simulink model "ModelMCC"  (R2018a)
settings: Solver=VariableStepAuto  StartTime=0.0  StopTime=10  RelTol=1e-3
undefined symbols (not defined in the file): A, f, J, K, L, N, R
libraries: simulink x1, powerlib x1
settings Model: Creator=Utilisateur  LastModifiedBy=Utilisateur

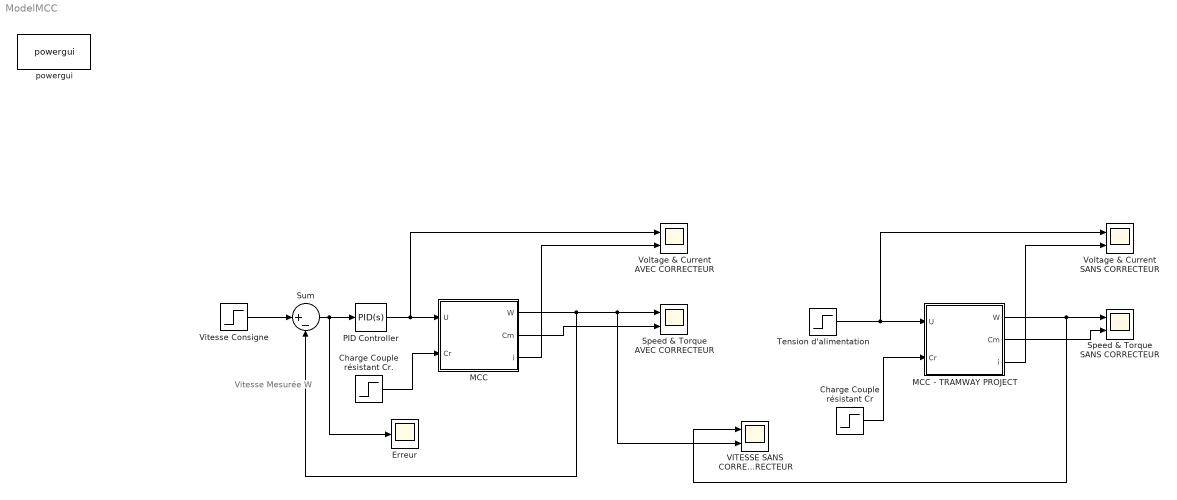
== system ModelMCC ==
  note: Vitesse Mesurée
      | W
  Charge Couple résistant Cr : Step  Time=5  After=30  SampleTime=0
  Charge Couple résistant Cr. : Step  Time=5  After=30  SampleTime=0
  Erreur : Scope
  MCC : Subsystem
  MCC - TRAMWAY PROJECT : Subsystem
  PID Controller : simulink/Continuous/PID Controller  Controller=PID  TimeDomain=Continuous-time  SampleTime=-1  IntegratorMethod=Forward Euler  FilterMethod=Forward Euler  Form=Parallel  UseFilter=on  ControllerParametersSource=internal  P=23.9565323270696  I=104.937795909472  D=-0.463662749906511  N=7.82954211558253  InitialConditionSource=internal  InitialConditionForIntegrator=0  InitialConditionForFilter=0  ExternalReset=none  LimitOutput=off  UpperSaturationLimit=inf  LowerSaturationLimit=-inf  LinearizeAsGain=on  AntiWindupMode=none  Kb=1  TrackingMode=off  Kt=1  PParamMin=[]  PParamMax=[]  IParamMin=[]  IParamMax=[]  DParamMin=[]  DParamMax=[]  NParamMin=[]  NParamMax=[]  KbParamMin=[]  KbParamMax=[]  KtParamMin=[]  KtParamMax=[]  POutMin=[]  POutMax=[]  IOutMin=[]  IOutMax=[]  DOutMin=[]  DOutMax=[]  NOutMin=[]  NOutMax=[]  KbOutMin=[]  KbOutMax=[]  KtOutMin=[]  KtOutMax=[]  IntegratorOutMin=[]  IntegratorOutMax=[]  FilterOutMin=[]  FilterOutMax=[]  SumOutMin=[]  SumOutMax=[]  SumI1OutMin=[]  SumI1OutMax=[]  SumI2OutMin=[]  SumI2OutMax=[]  SumI3OutMin=[]  SumI3OutMax=[]  SumDOutMin=[]  SumDOutMax=[]  SaturationOutMin=[]  SaturationOutMax=[]  IntegratorContinuousStateAttributes=''  IntegratorStateMustResolveToSignalObject=off  IntegratorRTWStateStorageClass=Auto  FilterContinuousStateAttributes=''  FilterStateMustResolveToSignalObject=off  FilterRTWStateStorageClass=Auto  DifferentiatorICPrevScaledInput=0  DifferentiatorOutMin=[]  DifferentiatorOutMax=[]  FilterDiffOutCoefMin=[]  FilterDiffOutCoefMax=[]  SumDenOutMin=[]  SumDenOutMax=[]  SumNumOutMin=[]  SumNumOutMax=[]  ReciprocalOutMin=[]  ReciprocalOutMax=[]  DivideOutMin=[]  DivideOutMax=[]  TunerSelectOption=Transfer Function Based (PID Tuner App)
  "Speed & Torque AVEC CORRECTEUR " : Scope  NumInputPorts=2
  Speed & Torque SANS CORRECTEUR : Scope  NumInputPorts=2
  Sum : Sum  Inputs=|+-
  Tension d'alimentation : Step  Time=0  After=30  SampleTime=0
  VITESSE SANS CORRECTEUR VITESSE AVEC CORRECTEUR : Scope  NumInputPorts=2
  Vitesse Consigne : Step  Time=0  After=2  SampleTime=0
  Voltage & Current AVEC CORRECTEUR : Scope  NumInputPorts=2
  Voltage & Current SANS CORRECTEUR : Scope  NumInputPorts=2
  powergui : powerlib/powergui  Priority=1  SimulationMode=Continuous  SampleTime=50e-6  frequency=60  Iterations=50  frequencyindice=60  Pbase=100e6  ErrMax=1e-4  UnitsV=kV  UnitsW=MW  buscounter=0  FunctionMessages=off  echomessages=off  EnableUseOfTLC=off  CurrentSourceSwitches=off  DisableSnubberDevices=off  DisableRonSwitches=off  DisableVfSwitches=off  DisplayEquations=off  SolverType=Tustin/Backward Euler (TBE)  Interpol=off  ExternalGateDelay=off  methode=off  Ts=100  x0status=blocks  SPID=on  SwTol=0  HookPort=off  RestoreLinks=warning  ResistiveCurrentMeasurement=off  Frange=[0:2:500]  Ylog=off  Xlog=on  ShowGrid=off  save=off  variable=ZData  structure=0  ZoomFFT=off  StartTime=0.0  cycles=1  DisplayStyle=1  fundamental=60  FreqAxis=off  MaxFrequency=1000  frequencyindicesteady=1  RmsSteady=1  display=off
  wires:
  MCC/2("Cm ") -> "Speed & Torque AVEC CORRECTEUR "/2
  MCC/3("i ") -> Voltage & Current AVEC CORRECTEUR/2
  Sum/1 -> Erreur/1, PID Controller/1
  Vitesse Consigne/1 -> Sum/1
  MCC/1(W) -> VITESSE SANS CORRECTEUR VITESSE AVEC CORRECTEUR/2, "Speed & Torque AVEC CORRECTEUR "/1, Sum/2
  PID Controller/1 -> Voltage & Current AVEC CORRECTEUR/1, MCC/1(U)
  MCC - TRAMWAY PROJECT/3("i ") -> Voltage & Current SANS CORRECTEUR/2
  MCC - TRAMWAY PROJECT/1(W) -> VITESSE SANS CORRECTEUR VITESSE AVEC CORRECTEUR/1, Speed & Torque SANS CORRECTEUR/1
  MCC - TRAMWAY PROJECT/2("Cm ") -> Speed & Torque SANS CORRECTEUR/2
  Charge Couple résistant Cr/1 -> MCC - TRAMWAY PROJECT/2(Cr)
  Tension d'alimentation/1 -> Voltage & Current SANS CORRECTEUR/1, MCC - TRAMWAY PROJECT/1(U)
  Charge Couple résistant Cr./1 -> MCC/2(Cr)

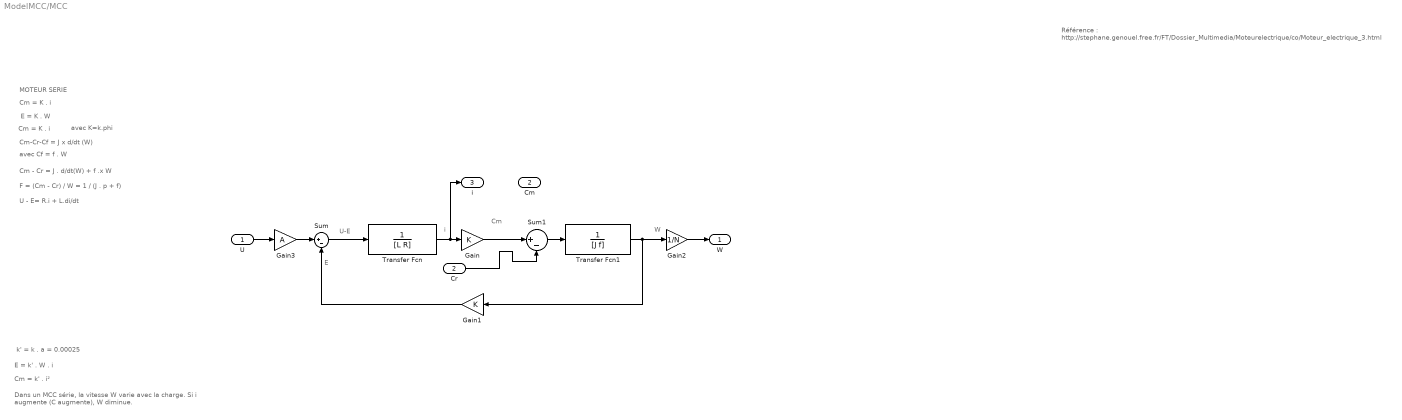
== system ModelMCC/MCC ==
  note: Référence : http://stephane.genouel.free.fr/FT/Dossier_Multimedia/Moteurelectrique/co/Moteur_electrique_3.html
  note: Dans un MCC série, la vitesse W varie avec la charge.
      | Si i augmente (C augmente), W diminue.
  note: MOTEUR SERIE
  note: avec K=k.phi
  note: U-E
  note: E
  note: W
  note: Cm
  note: i
  note: Cm-Cr-Cf = J x d/dt (W)
  note: Cm - Cr = J . d/dt(W) + f .x W
  note: F = (Cm - Cr) / W = 1 / (J . p + f)
  note: E = K . W
  note: Cm = K . i
  note: avec Cf = f . W
  note: Cm = K . i
  note: U - E= R.i + L.di/dt
  note: k' = k . a = 0.00025
  note: E = k' . W . i
  note: Cm = k' . i²
  U : Inport
  Cr : Inport  Port=2
  Gain : Gain  Gain=K
  Gain1 : Gain  Gain=K
  Gain2 : Gain  Gain=1/N
  Gain3 : Gain  Gain=A
  Sum : Sum  Inputs=|+-
  Sum1 : Sum  Inputs=|+-
  Transfer Fcn : TransferFcn  Denominator=[L R]
  Transfer Fcn1 : TransferFcn  Denominator=[J f]
  W : Outport
  "Cm " : Outport  Port=2
  "i " : Outport  Port=3
  wires:
  Sum1/1 -> Transfer Fcn1/1
  Gain/1 -> Sum1/1
  Cr/1 -> Sum1/2
  Transfer Fcn/1 -> "i "/1, Gain/1
  Sum/1 -> Transfer Fcn/1
  Gain2/1 -> W/1
  Transfer Fcn1/1 -> Gain2/1, Gain1/1
  Gain1/1 -> Sum/2
  U/1 -> Gain3/1
  Gain3/1 -> Sum/1

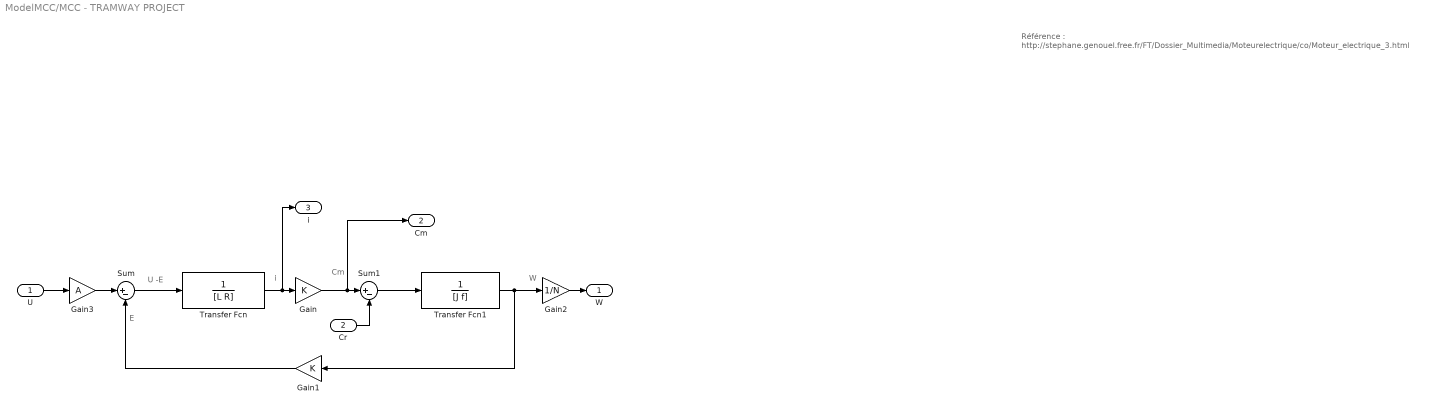
== system ModelMCC/MCC - TRAMWAY PROJECT ==
  note: Référence : http://stephane.genouel.free.fr/FT/Dossier_Multimedia/Moteurelectrique/co/Moteur_electrique_3.html
  note: U -E
  note: E
  note: W
  note: Cm
  note: i
  U : Inport
  Cr : Inport  Port=2
  Gain : Gain  Gain=K
  Gain1 : Gain  Gain=K
  Gain2 : Gain  Gain=1/N
  Gain3 : Gain  Gain=A
  Sum : Sum  Inputs=|+-
  Sum1 : Sum  Inputs=|+-
  Transfer Fcn : TransferFcn  Denominator=[L R]
  Transfer Fcn1 : TransferFcn  Denominator=[J f]
  W : Outport
  "Cm " : Outport  Port=2
  "i " : Outport  Port=3
  wires:
  Gain/1 -> "Cm "/1, Sum1/1
  Cr/1 -> Sum1/2
  Transfer Fcn/1 -> "i "/1, Gain/1
  Sum/1 -> Transfer Fcn/1
  Gain2/1 -> W/1
  Transfer Fcn1/1 -> Gain2/1, Gain1/1
  Gain1/1 -> Sum/2
  U/1 -> Gain3/1
  Gain3/1 -> Sum/1
  Sum1/1 -> Transfer Fcn1/1
